simulink model "SimForces2022a"  (R2022a)
settings: Solver=daessc  StartTime=0.0  StopTime=10  FixedStep=0.001  RelTol=1e-4
values from neighbouring files (symbols this model uses):
  Bc1_V = [0;0;0;0;0;0]    [initializeSimulationGP.m]
  D22F = [0;0;0;0;0;0]    [initializeSimulationGP.m]
  filtDV = init2ndOrderLowPassFilter(35*2*pi,1,controller.dT)    [initializeLowPassFilters.m]
  filtEnc = init2ndOrderLowPassFilter(35*2*pi,1,controller.dT)    [initializeLowPassFilters.m]
undefined symbols (not defined in the file or in its folder): aux, B11_r_B11Tc1, B11_V, B11Ftot, B12_r_B12Tc2, B12_Rot_Tc2, B12_U_Tc2, B12_V, B12Ftot, B31_r_B31B41, B31_V, B31FTot, B32_r_B32B42, B32_Rot_B42, B32_U_B42, B32_V, B32FTot, B41_r_B41Tc1, B41_V, B41FTot, B42_r_B42Tc2, B42_Rot_Tc2, B42_U_Tc2, B42_V, B42FTot, B52_r_B52P32, B52_Rot_P32, B52_U_P32, B52_V, B52Ftot, Bc1_r_Bc1B11, Bc1_r_Bc1B31, Bc1FTot, Bc2_r_Bc2B12, Bc2_r_Bc2B32, Bc2_Rot_B12, Bc2_Rot_B32, Bc2_U_B12, Bc2_U_B32, Bc2_V, Bc2Tot, controller, cyl1, cyl2, D22_V, dq1, dq11, dq12, dq2, dq21, dq22, dx1, dx2, dxt2, fc1, fc1r, fc2, fc2r, fct2, fct2r ... (+61)
libraries: sm_lib x32, nesl_utility x20
(part 1 of 7)
settings Model: Creator=liikaneh  LastModifiedBy=casey
settings SolverCC: AlgebraicLoopSolver=TrustRegion
settings OptimizationCC: DefaultParameterBehavior=Inlined  GainParamInheritBuiltInType=on  UseFloatMulNetSlope=on  InlineInvariantSignals=on  EfficientFloat2IntCast=on
settings DebuggingCC: ReadBeforeWriteMsg=DisableAll  WriteAfterWriteMsg=DisableAll  WriteAfterReadMsg=DisableAll  MultiTaskDSMMsg=none  UnconnectedInputMsg=warning  UnconnectedOutputMsg=warning  UnconnectedLineMsg=warning  SFMachineParentedDataDiag=warning  ArithmeticOperatorsInVariantConditions=warning
settings ModelReferenceCC: UpdateModelReferenceTargets=IfOutOfDate
settings SFSimCC: SFSimEcho=off  SimUseLocalCustomCode=off  CustomCodeUndefinedFunction=UseInterfaceOnly
settings RTWCC: RTWUseLocalCustomCode=off  BuildConfiguration=Faster Runs  DLArmComputeVersion=19.05
settings GRTTargetCC: MatFileLogging=off  SupportNonFinite=off
settings DiagnosticsConfigSet: SimMechanicsRigidlyBoundBlock=none

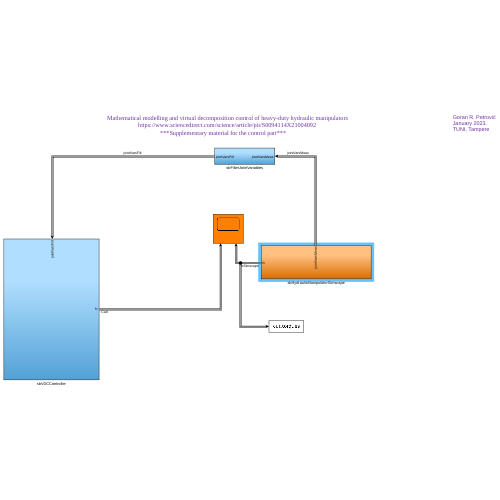
[thumbnail: Simulink's stored preview of the top-level diagram]
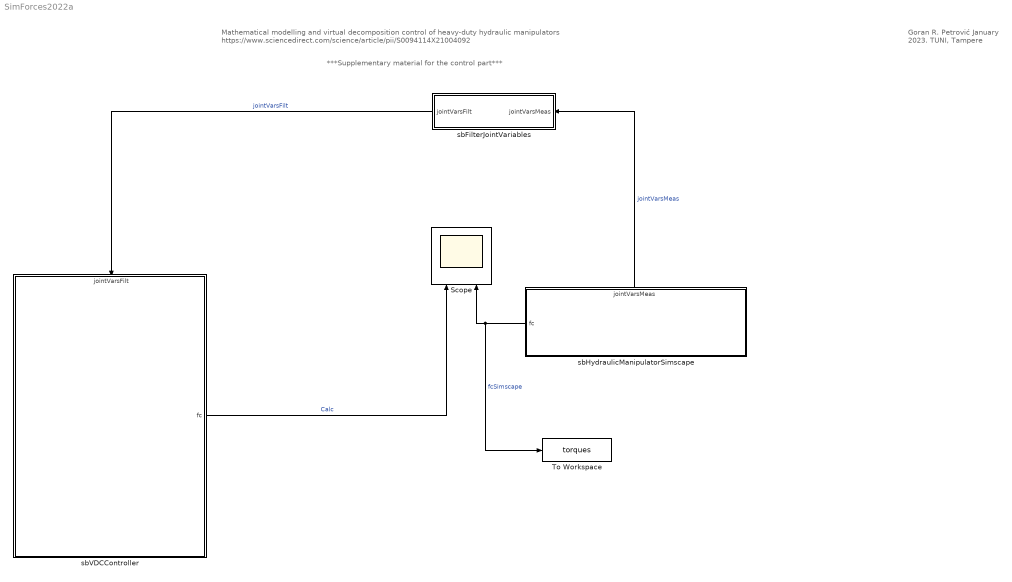
== system SimForces2022a ==
  note: ***Supplementary material for the control part***
  note: Mathematical modelling and virtual decomposition control of heavy-duty hydraulic manipulators
      | https://www.sciencedirect.com/science/article/pii/S0094114X21004092
  note: Goran R. Petrović
      | January 2023.
      | TUNI, Tampere
  Scope : Scope  NumInputPorts=2
  To Workspace : ToWorkspace  VariableName=torques  SaveFormat=Timeseries  SampleTime=-1
  sbFilterJointVariables : Subsystem
  sbHydraulicManipulatorSimscape : Subsystem
      settings: PortSchema="{\"entries\":[{\"content\":{\"sides\":[{\"content\":{\"connectorIds\":[\"Out2\"]},\"type\":\"ConnectorPlacement.EquallySpacedRectSide\",\"uuid\":\"f7b00952-2d51-484f-abea-a7edf7f1803a\"},{\"content\":{\"connectorIds\":[],\"side\":\"RIGHT\"},\"type\":\"ConnectorPlacement.EquallySpacedRectSide\",\"uuid\":\"cec57a8d-f407-43fc-b54f-695abbd67ebc\"},{\"content\":{\"connectorIds\":[\"Out1\"],\"side\":\"TOP\"},\"type\":\"ConnectorPlacement.EquallySpacedRectSide\",\"uuid\":\"36c8b0b2-f27a-4d8c-8e2c-18a80d711d3e\"}]},\"type\":\"ConnectorPlacement.EquallySpacedConnector\",\"uuid\":\"9ce8286e-5e91-4ec7-b364-968722180a48\"}],\"packageUris\":[\"http://schema.mathworks.com/mf0/Connector/R2020b\"],\"version\":\"1.0\"}"
  sbVDCController : Subsystem
      settings: PortSchema="{\"entries\":[{\"content\":{\"sides\":[{\"content\":{\"connectorIds\":[]},\"type\":\"ConnectorPlacement.EquallySpacedRectSide\",\"uuid\":\"7b05da7d-8e98-4260-b965-883aeff80f6d\"},{\"content\":{\"connectorIds\":[\"Out1\"],\"side\":\"RIGHT\"},\"type\":\"ConnectorPlacement.EquallySpacedRectSide\",\"uuid\":\"bab503f6-0cf2-4d25-8612-166524dadf44\"},{\"content\":{\"connectorIds\":[\"In1\"],\"side\":\"TOP\"},\"type\":\"ConnectorPlacement.EquallySpacedRectSide\",\"uuid\":\"dc9bf139-dfcc-4316-b9ab-c299ea19db13\"}]},\"type\":\"ConnectorPlacement.EquallySpacedConnector\",\"uuid\":\"a723f5e0-c36b-4f3a-b452-df4ada5825ab\"}],\"packageUris\":[\"http://schema.mathworks.com/mf0/Connector/R2020b\"],\"version\":\"1.0\"}"
  wires:
  sbHydraulicManipulatorSimscape/1(jointVarsMeas) -> sbFilterJointVariables/1(jointVarsMeas)  "jointVarsMeas"
  sbFilterJointVariables/1(jointVarsFilt) -> sbVDCController/1(jointVarsFilt)  "jointVarsFilt"
  sbVDCController/1(fc) -> Scope/1  "Calc"
  sbHydraulicManipulatorSimscape/2(fc) -> To Workspace/1, Scope/2  "fcSimscape"

== system SimForces2022a/sbFilterJointVariables ==
  jointVarsMeas : Inport  OutDataTypeStr=double  PortDimensions=3  SampleTime=controller.dT
  Bus Creator : BusCreator  Inputs=theta1Filt,theta2Filt,xt2Filt
  Bus Selector : BusSelector  OutputSignals=theta1Meas,theta2Meas,xt2Meas
  sbTheta1LowPassFilter : Subsystem
  sbTheta2LowPassFilter : Subsystem
  sbxt2LowPassFilter : Subsystem
  jointVarsFilt : Outport  OutDataTypeStr=double  PortDimensions=3  SampleTime=controller.dT
  wires:
  sbxt2LowPassFilter/1(xt2Filt) -> Bus Creator/3  "xt2Filt"
  sbTheta2LowPassFilter/1(theta2Filt) -> Bus Creator/2  "theta2Filt"
  sbTheta1LowPassFilter/1(theta1Filt) -> Bus Creator/1  "theta1Filt"
  Bus Selector/2 -> sbTheta2LowPassFilter/1(theta2Meas)  "<theta2Meas>"
  Bus Selector/1 -> sbTheta1LowPassFilter/1(theta1Meas)  "<theta1Meas>"
  Bus Selector/3 -> sbxt2LowPassFilter/1(xt2Meas)  "<xt2Meas>"
  jointVarsMeas/1 -> Bus Selector/1
  Bus Creator/1 -> jointVarsFilt/1

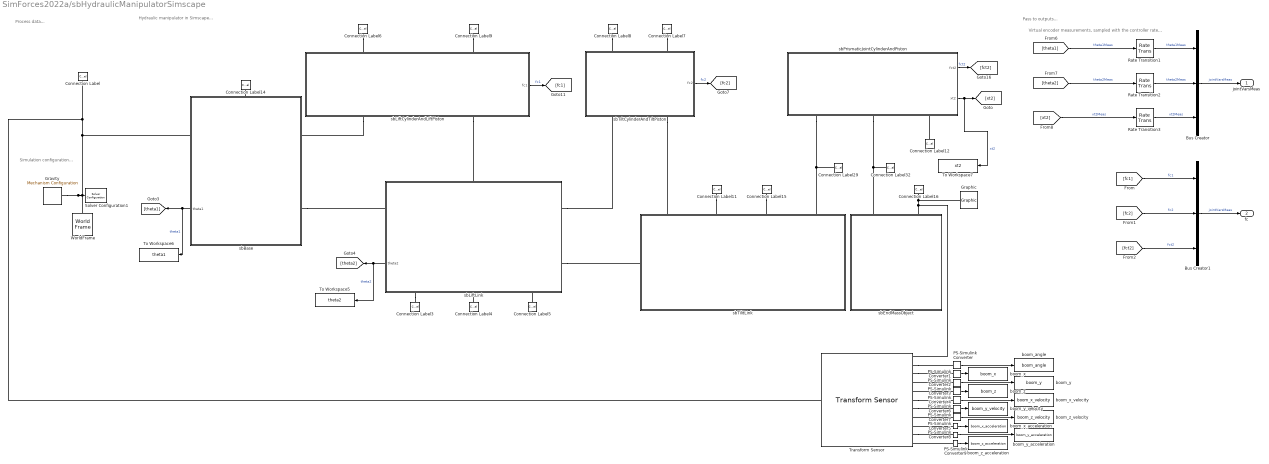
== system SimForces2022a/sbHydraulicManipulatorSimscape ==
  note: Process data...
  note: Hydraulic manipulator in Simscape...
  note: Simulation configuration...
  note: Pass to outputs...
  note: Virtual encoder measurements, sampled with the controller rate...
  Bus Creator : BusCreator  Inputs=theta1Meas,theta2Meas,xt2Meas
  Bus Creator1 : BusCreator  Inputs=fc1,fc2,fct2
  Connection Label : ConnectionLabel  Label=W
  Connection Label11 : ConnectionLabel  Label=B12
  Connection Label12 : ConnectionLabel  Label=B52
  Connection Label14 : ConnectionLabel  Label=Bc1
  Connection Label15 : ConnectionLabel  Label=Tc2
  Connection Label16 : ConnectionLabel  Label=D22
  Connection Label29 : ConnectionLabel  Label=P22
  Connection Label3 : ConnectionLabel  Label=Tc1
  Connection Label32 : ConnectionLabel  Label=P32
  Connection Label4 : ConnectionLabel  Label=B11
  Connection Label5 : ConnectionLabel  Label=Bc2
  Connection Label6 : ConnectionLabel  Label=B31
  Connection Label7 : ConnectionLabel  Label=B42
  Connection Label8 : ConnectionLabel  Label=B32
  Connection Label9 : ConnectionLabel  Label=B41
  Graphic : sm_lib/Body Elements/Graphic  GraphicType=Marker  MarkerShape=Frame  MarkerSize=50  GraphicVisPropType=SimpleVisualProperties  GraphicDiffuseColor=[0.9294 0.6941 0.1255]  GraphicSpecularColor=[0.5 0.5 0.5 1.0]  GraphicAmbientColor=[0.15 0.15 0.15 1.0]  GraphicEmissiveColor=[0.0 0.0 0.0 1.0]  GraphicShininess=75  GraphicOpacity=1.0
  Gravity : sm_lib/Utilities/Mechanism Configuration  UniformGravity=Constant  GravityVector=-gravity.Wg  GravityUnits=m/s^2  LinearizationDelta=0.001  JointModeTransitionNonlinearIterations=2
  PS-Simulink Converter{,1..9} (10 alike) : nesl_utility/PS-Simulink Converter  PhysicalDomain=network_engine_domain  SubClassName=ps_output  LeftPortType=input  RightPortType=output  PseudoPeriodic=off  Frequencies=[]  VectorFormat=inherit  Unit=inherit  AffineConversion=off
      settings: SourceProductBaseCode=SS,PW,VE
  Rate Transition1 : RateTransition  InitialCondition=initVals.theta10  OutPortSampleTime=controller.dT
  Rate Transition2 : RateTransition  InitialCondition=initVals.theta20  OutPortSampleTime=controller.dT
  Rate Transition3 : RateTransition  InitialCondition=initVals.xt20  OutPortSampleTime=controller.dT
  Solver Configuration1 : nesl_utility/Solver Configuration  PhysicalDomain=network_engine_domain  SubClassName=solver  LeftPortType=input  RightPortType=generic  Tones=[]  Harmonics=[]  SimulateNoise=off  Profile=off  UseLocalSampling=off  EnableSwitchedLinearOptims=on  FrequencyDomain=off  UseCCode=off  RelTol=0.001  AbsTol=1e-06  MinStep=1e-09  ToWorkspace=off  RevertToSquareIcSolve=off  NumHomotopyIterations=100  PhasorMode=off  PhasorModeNumHarmonics=1  IndexReductionMethod=DerivativeReplacement  DoDC=on  ResidualTolerance=1e-9  UseLocalSolver=off  LocalSolverChoice=NE_TRAPEZOIDAL_ADVANCER  LocalSolverSampleTime=0.002  DoFixedCost=off  MaxNonlinIter=3  MaxModeIter=2  ComputeImpulses=off  ImpulseIterations=2  LinearAlgebra=Sparse  LinearAlgebraNumThread=0  EquationFormulation=NE_TIME_EF  DelaysMemoryBudget=1024  AutomaticFiltering=on  FilteringTimeConstant=0.001  PartitionStorageMethod=AS_NEEDED  PartitionMemoryBudget=1024  PartitionMethod=FAST
      settings: SourceProductBaseCode=SS,PW,VE
  To Workspace5 : ToWorkspace  VariableName=theta2  SaveFormat=Timeseries  SampleTime=-1
  To Workspace6 : ToWorkspace  VariableName=theta1  SaveFormat=Timeseries  SampleTime=-1
  To Workspace7 : ToWorkspace  VariableName=xt2  SaveFormat=Timeseries  SampleTime=-1
  Transform Sensor : sm_lib/Frames and Transforms/Transform Sensor  MeasurementFrame=World  SenseAngle=on  SenseAxis=off  SenseAngle1=off  SenseAngle2=off  SenseAngle3=off  SenseQ=off  SenseR=off  SenseOmegaX=off  SenseOmegaY=off  SenseOmegaZ=off  SenseOmega1=off  SenseOmega2=off  SenseOmega3=off  SenseQDot=off  SenseRDot=off  SenseAlphaX=off  SenseAlphaY=off  SenseAlphaZ=off  SenseAlpha1=off  SenseAlpha2=off  SenseAlpha3=off  SenseQDDot=off  SenseRDDot=off  SenseX=on  SenseY=on  SenseZ=on  SenseRad=off  SenseAzim=off  SenseDist=off  SenseInc=off  SenseXDot=on  SenseYDot=on  SenseZDot=on  SenseRadDot=off  SenseAzimDot=off  SenseDistDot=off  SenseIncDot=off  SenseXDDot=on  SenseYDDot=on  SenseZDDot=on  SenseRadDDot=off  SenseAzimDDot=off  SenseDistDDot=off  SenseIncDDot=off
  WorldFrame : sm_lib/Frames and Transforms/World Frame
  boom_angle : ToWorkspace  VariableName=boom_angle  SaveFormat=Structure  SampleTime=-1
      settings: Save2DSignal=2-D array (concatenate along first dimension)
  boom_x : ToWorkspace  VariableName=boom_x  SaveFormat=Structure With Time  SampleTime=-1
  boom_x_acceleration : ToWorkspace  VariableName=boom_x_acceleration  SaveFormat=Structure  SampleTime=-1
      settings: Save2DSignal=2-D array (concatenate along first dimension)
  boom_x_velocity : ToWorkspace  VariableName=boom_x_velocity  SaveFormat=Structure  SampleTime=-1
      settings: Save2DSignal=2-D array (concatenate along first dimension)
  boom_y : ToWorkspace  VariableName=boom_y  SaveFormat=Structure  SampleTime=-1
      settings: Save2DSignal=2-D array (concatenate along first dimension)
  boom_y_acceleration : ToWorkspace  VariableName=boom_y_acceleration  SaveFormat=Structure  SampleTime=-1
      settings: Save2DSignal=2-D array (concatenate along first dimension)
  boom_y_velocity : ToWorkspace  VariableName=boom_y_velocity  SaveFormat=Structure  SampleTime=-1
      settings: Save2DSignal=2-D array (concatenate along first dimension)
  boom_z : ToWorkspace  VariableName=boom_z  SaveFormat=Structure  SampleTime=-1
      settings: Save2DSignal=2-D array (concatenate along first dimension)
  boom_z_acceleration : ToWorkspace  VariableName=boom_z_acceleration  SaveFormat=Structure  SampleTime=-1
      settings: Save2DSignal=2-D array (concatenate along first dimension)
  boom_z_velocity : ToWorkspace  VariableName=boom_z_velocity  SaveFormat=Structure  SampleTime=-1
      settings: Save2DSignal=2-D array (concatenate along first dimension)
  sbBase : Subsystem
      settings: PortSchema="{\"entries\":[{\"content\":{\"sides\":[{\"content\":{\"connectorIds\":[\"LConn1\",\"Out1\"]},\"type\":\"ConnectorPlacement.EquallySpacedRectSide\",\"uuid\":\"74e7f3c6-cbce-4102-a556-47a2132f5eea\"},{\"content\":{\"connectorIds\":[\"RConn1\",\"RConn2\"],\"side\":\"RIGHT\"},\"type\":\"ConnectorPlacement.EquallySpacedRectSide\",\"uuid\":\"9dc74751-c8ff-4cb6-874a-dcd58e00de96\"},{\"content\":{\"connectorIds\":[\"LConn2\"],\"side\":\"TOP\"},\"type\":\"ConnectorPlacement.EquallySpacedRectSide\",\"uuid\":\"06e145de-a8a9-4531-940d-434d89c78f5b\"}]},\"type\":\"ConnectorPlacement.EquallySpacedConnector\",\"uuid\":\"f796a1f4-9531-411f-8f55-fdef488b8a52\"}],\"packageUris\":[\"http://schema.mathworks.com/mf0/Connector/R2020b\"],\"version\":\"1.0\"}"
  sbEndMassObject : Subsystem
      settings: PortSchema="{\"entries\":[{\"content\":{\"sides\":[{\"content\":{\"connectorIds\":[]},\"type\":\"ConnectorPlacement.EquallySpacedRectSide\",\"uuid\":\"c1652833-a888-40a4-a60e-17be9708feae\"},{\"content\":{\"connectorIds\":[],\"side\":\"RIGHT\"},\"type\":\"ConnectorPlacement.EquallySpacedRectSide\",\"uuid\":\"55671429-adc4-418e-b6f5-c624f049c776\"},{\"content\":{\"connectorIds\":[\"LConn1\",\"LConn2\"],\"side\":\"TOP\"},\"type\":\"ConnectorPlacement.EquallySpacedRectSide\",\"uuid\":\"549e793d-1b28-4f93-9706-f4524b8bc4e2\"}]},\"type\":\"ConnectorPlacement.EquallySpacedConnector\",\"uuid\":\"9a6e434f-5824-411f-a3a4-9b8ec603a501\"}],\"packageUris\":[\"http://schema.mathworks.com/mf0/Connector/19700101\"],\"version\":\"1.0\"}"
  sbLiftCylinderAndLiftPiston : Subsystem
      settings: PortSchema="{\"entries\":[{\"content\":{\"sides\":[{\"content\":{\"connectorIds\":[]},\"type\":\"ConnectorPlacement.EquallySpacedRectSide\",\"uuid\":\"a609877c-275e-4024-96c6-67831631fbf9\"},{\"content\":{\"connectorIds\":[\"Out1\"],\"side\":\"RIGHT\"},\"type\":\"ConnectorPlacement.EquallySpacedRectSide\",\"uuid\":\"b747ace3-04d7-42f4-87a7-c62fd6093e0d\"},{\"content\":{\"connectorIds\":[\"LConn1\",\"LConn2\"],\"side\":\"TOP\"},\"type\":\"ConnectorPlacement.EquallySpacedRectSide\",\"uuid\":\"5f9db8d6-814e-4333-b197-0e9dcf847d3e\"},{\"content\":{\"connectorIds\":[\"RConn1\",\"RConn2\"],\"side\":\"BOTTOM\"},\"type\":\"ConnectorPlacement.EquallySpacedRectSide\",\"uuid\":\"d1d564c3-4146-4330-9936-8dd25e0cb4bf\"}]},\"type\":\"ConnectorPlacement.EquallySpacedConnector\",\"uuid\":\"d00f43c3-717c-4aa5-b919-dd57ad6708f7\"}],\"packageUris\":[\"http://schema.mathworks.com/mf0/Connector/R2020b\"],\"version\":\"1.0\"}"
  sbLiftLink : Subsystem
      settings: PortSchema="{\"entries\":[{\"content\":{\"sides\":[{\"content\":{\"connectorIds\":[\"LConn1\",\"LConn2\"]},\"type\":\"ConnectorPlacement.EquallySpacedRectSide\",\"uuid\":\"50668ed3-3246-41c6-a320-c5b34ebd86b6\"},{\"content\":{\"connectorIds\":[\"RConn1\",\"Out1\"],\"side\":\"RIGHT\"},\"type\":\"ConnectorPlacement.EquallySpacedRectSide\",\"uuid\":\"d76ddc23-e4dc-4bdf-9e15-3eadac6cf1e2\"},{\"content\":{\"connectorIds\":[\"LConn3\"],\"side\":\"TOP\"},\"type\":\"ConnectorPlacement.EquallySpacedRectSide\",\"uuid\":\"5458eee7-805c-4d74-888c-3f811d80880c\"},{\"content\":{\"connectorIds\":[\"RConn2\",\"RConn3\",\"RConn4\"],\"side\":\"BOTTOM\"},\"type\":\"ConnectorPlacement.EquallySpacedRectSide\",\"uuid\":\"6f630415-b321-44c9-a6f9-9daa6b5086dd\"}]},\"type\":\"ConnectorPlacement.EquallySpacedConnector\",\"uuid\":\"adbb0eba-5908-47e0-8cde-3ca3a2901b66\"}],\"packageUris\":[\"http://schema.mathworks.com/mf0/Connector/R2020b\"],\"version\":\"1.0\"}"
  sbPrismaticJointCylinderAndPiston : Subsystem
      settings: PortSchema="{\"entries\":[{\"content\":{\"sides\":[{\"content\":{\"connectorIds\":[]},\"type\":\"ConnectorPlacement.EquallySpacedRectSide\",\"uuid\":\"002196eb-b81c-4ad4-9df1-33c4ef5d5c77\"},{\"content\":{\"connectorIds\":[\"Out1\",\"Out2\"],\"side\":\"RIGHT\"},\"type\":\"ConnectorPlacement.EquallySpacedRectSide\",\"uuid\":\"e0d61efe-ea5d-4756-bea5-1d107b09975a\"},{\"content\":{\"connectorIds\":[],\"side\":\"TOP\"},\"type\":\"ConnectorPlacement.EquallySpacedRectSide\",\"uuid\":\"1a952641-c922-4f91-9854-1cf1d6e715db\"},{\"content\":{\"connectorIds\":[\"RConn1\",\"RConn2\",\"RConn3\"],\"side\":\"BOTTOM\"},\"type\":\"ConnectorPlacement.EquallySpacedRectSide\",\"uuid\":\"13c3128f-85d9-4df5-9ae2-f45a9cb5a20e\"}]},\"type\":\"ConnectorPlacement.EquallySpacedConnector\",\"uuid\":\"7bd12321-8448-494e-b8ce-fe2f63fec7f7\"}],\"packageUris\":[\"http://schema.mathworks.com/mf0/Connector/R2020b\"],\"version\":\"1.0\"}"
  sbTilitLink : Subsystem
      settings: PortSchema="{\"entries\":[{\"content\":{\"sides\":[{\"content\":{\"connectorIds\":[]},\"type\":\"ConnectorPlacement.EquallySpacedRectSide\",\"uuid\":\"3124f0ed-3daa-4e61-aa81-877c0a0fd3a0\"},{\"content\":{\"connectorIds\":[\"RConn1\"],\"side\":\"RIGHT\"},\"type\":\"ConnectorPlacement.EquallySpacedRectSide\",\"uuid\":\"bc27bd78-7de5-476c-8b4b-17e2ed4c2476\"},{\"content\":{\"connectorIds\":[\"LConn1\",\"LConn2\",\"LConn3\",\"LConn4\"],\"side\":\"TOP\"},\"type\":\"ConnectorPlacement.EquallySpacedRectSide\",\"uuid\":\"46b542cf-bb62-4410-9418-b726c84ee3f9\"}]},\"type\":\"ConnectorPlacement.EquallySpacedConnector\",\"uuid\":\"3938a7f2-fa69-42c9-abcf-1c8c25e9b66f\"}],\"packageUris\":[\"http://schema.mathworks.com/mf0/Connector/19700101\"],\"version\":\"1.0\"}"
  sbTiltCylinderAndTiltPiston : Subsystem
      settings: PortSchema="{\"entries\":[{\"content\":{\"sides\":[{\"content\":{\"connectorIds\":[]},\"type\":\"ConnectorPlacement.EquallySpacedRectSide\",\"uuid\":\"a609877c-275e-4024-96c6-67831631fbf9\"},{\"content\":{\"connectorIds\":[\"Out1\"],\"side\":\"RIGHT\"},\"type\":\"ConnectorPlacement.EquallySpacedRectSide\",\"uuid\":\"b747ace3-04d7-42f4-87a7-c62fd6093e0d\"},{\"content\":{\"connectorIds\":[\"LConn1\",\"LConn2\"],\"side\":\"TOP\"},\"type\":\"ConnectorPlacement.EquallySpacedRectSide\",\"uuid\":\"5f9db8d6-814e-4333-b197-0e9dcf847d3e\"},{\"content\":{\"connectorIds\":[\"RConn1\",\"RConn2\"],\"side\":\"BOTTOM\"},\"type\":\"ConnectorPlacement.EquallySpacedRectSide\",\"uuid\":\"d1d564c3-4146-4330-9936-8dd25e0cb4bf\"}]},\"type\":\"ConnectorPlacement.EquallySpacedConnector\",\"uuid\":\"d00f43c3-717c-4aa5-b919-dd57ad6708f7\"}],\"packageUris\":[\"http://schema.mathworks.com/mf0/Connector/R2020b\"],\"version\":\"1.0\"}"
  jointVarsMeas : Outport
  fc : Outport  Port=2
  wires:
  sbLiftCylinderAndLiftPiston/1(fc1) -> [fc1]  "fc1"
  sbTiltCylinderAndTiltPiston/1(fc2) -> [fc2]  "fc2"
  sbPrismaticJointCylinderAndPiston/1(fct2) -> [fct2]  "fct2"
  sbLiftLink/1(theta2) -> [theta2], To Workspace5/1  "theta2"
  sbBase/1(theta1) -> To Workspace6/1, [theta1]  "theta1"
  Bus Creator/1 -> jointVarsMeas/1  "jointVarsMeas"
  [theta2] -> Rate Transition2/1  "theta2Meas"
  Rate Transition1/1 -> Bus Creator/1  "theta1Meas"
  Rate Transition2/1 -> Bus Creator/2  "theta2Meas"
  Rate Transition3/1 -> Bus Creator/3  "xt2Meas"
  [theta1] -> Rate Transition1/1  "theta1Meas"
  [xt2] -> Rate Transition3/1  "xt2Meas"
  [fc1] -> Bus Creator1/1  "fc1"
  [fc2] -> Bus Creator1/2  "fc2"
  [fct2] -> Bus Creator1/3  "fct2"
  Bus Creator1/1 -> fc/1  "jointVarsMeas"
  sbPrismaticJointCylinderAndPiston/2(xt2) -> To Workspace7/1, [xt2]  "xt2"
  PS-Simulink Converter4/1 -> boom_x_velocity/1
  PS-Simulink Converter3/1 -> boom_z/1
  PS-Simulink Converter/1 -> boom_angle/1
  PS-Simulink Converter1/1 -> boom_x/1
  PS-Simulink Converter2/1 -> boom_y/1
  PS-Simulink Converter6/1 -> boom_y_velocity/1
  PS-Simulink Converter5/1 -> boom_x_acceleration/1
  PS-Simulink Converter7/1 -> boom_z_velocity/1
  PS-Simulink Converter8/1 -> boom_y_acceleration/1
  PS-Simulink Converter9/1 -> boom_z_acceleration/1
  connections:
  Gravity/RConn1 -- sbBase/LConn1 -- Connection Label/LConn1 -- Transform Sensor/LConn1 -- WorldFrame/RConn1 -- Solver Configuration1/RConn1
  sbLiftLink/LConn1 -- sbTiltCylinderAndTiltPiston/RConn1
  sbLiftLink/LConn2 -- sbTilitLink/RConn1
  sbTiltCylinderAndTiltPiston/RConn2 -- sbTilitLink/LConn4
  sbLiftCylinderAndLiftPiston/RConn2 -- sbLiftLink/LConn3
  sbBase/RConn2 -- sbLiftLink/RConn1
  sbLiftCylinderAndLiftPiston/RConn1 -- sbBase/RConn1
  sbLiftLink/RConn4 -- Connection Label3/LConn1
  Connection Label4/LConn1 -- sbLiftLink/RConn3
  Connection Label5/LConn1 -- sbLiftLink/RConn2
  Connection Label6/LConn1 -- sbLiftCylinderAndLiftPiston/LConn1
  Connection Label9/LConn1 -- sbLiftCylinderAndLiftPiston/LConn2
  Connection Label7/LConn1 -- sbTiltCylinderAndTiltPiston/LConn2
  Connection Label8/LConn1 -- sbTiltCylinderAndTiltPiston/LConn1
  Connection Label11/LConn1 -- sbTilitLink/LConn3
  Connection Label15/LConn1 -- sbTilitLink/LConn2
  Connection Label16/LConn1 -- Graphic/RConn1 -- sbEndMassObject/LConn2 -- Transform Sensor/RConn1
  Connection Label14/LConn1 -- sbBase/LConn2
  Connection Label12/LConn1 -- sbPrismaticJointCylinderAndPiston/RConn3
  sbPrismaticJointCylinderAndPiston/RConn1 -- Connection Label29/LConn1 -- sbTilitLink/LConn1
  sbPrismaticJointCylinderAndPiston/RConn2 -- sbEndMassObject/LConn1 -- Connection Label32/LConn1
  Transform Sensor/RConn2 -- PS-Simulink Converter/LConn1
  Transform Sensor/RConn3 -- PS-Simulink Converter1/LConn1
  PS-Simulink Converter2/LConn1 -- Transform Sensor/RConn4
  Transform Sensor/RConn6 -- PS-Simulink Converter4/LConn1
  PS-Simulink Converter3/LConn1 -- Transform Sensor/RConn5
  PS-Simulink Converter5/LConn1 -- Transform Sensor/RConn9
  Transform Sensor/RConn7 -- PS-Simulink Converter6/LConn1
  PS-Simulink Converter7/LConn1 -- Transform Sensor/RConn8
  Transform Sensor/RConn10 -- PS-Simulink Converter8/LConn1
  PS-Simulink Converter9/LConn1 -- Transform Sensor/RConn11

== system SimForces2022a/sbVDCController ==
  note: Extract actuator forces per (73) and (76).
  note: Forming total forces.
  note: Geometric relations (18) - (23), velocities (24) - (34), along with all the necessary rotation matrices and force/velocity
      | transformation matrices (5) are formed here.
  note: Calculate qj angles as they are starting point for kinematic relations (18) - (23).
  note: Required piston forces for comparison puroposes...
  note: Select from existing buses...
  note: No required force imposing on the surroundings...
  note: Zero-vector for a fixed base....
  note: Filtered values of joint variables...
  note: Process data...
  note: Get inputs...
  note: Pass to outputs...
  jointVarsFilt : Inport
  Bus Selector : BusSelector  OutputSignals=theta1Filt,theta2Filt,xt2Filt
  Constant1 : Constant  Value=Bc1_V
  D22F : Constant  Value=D22F
  Rate Transition : RateTransition  OutPortSampleTime=controller.dT
  sbAuxiliaryJointAngles : Subsystem
  sbCalculateRequiredActuatorForces : Subsystem
  sbFormAnalyticQuantities : Subsystem
  sbFormTotalRequiredForces : Subsystem
  fc : Outport
  wires:
  Bus Selector/3 -> [xt2Filt]  "<xt2Filt>"
  Bus Selector/2 -> [theta2Filt]  "<theta2Filt>"
  [Bc1V] -> sbFormAnalyticQuantities/4(Bc1V)  "Bc1V"
  [D22F] -> sbCalculateRequiredActuatorForces/4(D22F)  "D22F"
  sbAuxiliaryJointAngles/1(q1) -> [q1]  "q1"
  [xt2Filt] -> sbFormAnalyticQuantities/3(xt2Filt)  "xt2Filt"
  [jointVarsFilt] -> Bus Selector/1  "jointVarsFilt"
  [WRotX] -> sbFormTotalRequiredForces/2(WRotX)  "WRotX"
  sbFormTotalRequiredForces/1(FTotX) -> [FTotX]  "FTotX"
  [velsX] -> sbFormTotalRequiredForces/1(velsX)  "velsX"
  [FTotX] -> sbCalculateRequiredActuatorForces/1(FTotX)  "FTotX"
  [geomPropX] -> sbCalculateRequiredActuatorForces/3(geomPropX)  "geomPropX"
  Constant1/1 -> [Bc1V]  "Bc1_V"
  sbFormAnalyticQuantities/3(UMatsX) -> [UMatsX]  "UMatsX"
  sbFormAnalyticQuantities/1(geomPropX) -> [geomPropX]  "geomPropX"
  [theta2Filt] -> sbAuxiliaryJointAngles/2(theta2Filt)  "theta2Filt"
  [theta1Filt] -> sbAuxiliaryJointAngles/1(theta1Filt)  "theta1Filt"
  sbFormAnalyticQuantities/2(WRotX) -> [WRotX]  "WRotX"
  D22F/1 -> [D22F]  "D22F"
  [UMatsX] -> sbCalculateRequiredActuatorForces/2(UMatsX)  "UMatsX"
  [q2] -> sbFormAnalyticQuantities/2(q2)  "q2"
  [q1] -> sbFormAnalyticQuantities/1(q1)  "q1"
  sbAuxiliaryJointAngles/2(q2) -> [q2]  "q2"
  sbFormAnalyticQuantities/4(velsX) -> [velsX]  "velsX"
  Bus Selector/1 -> [theta1Filt]  "<theta1Filt>"
  jointVarsFilt/1 -> [jointVarsFilt]  "jointVarsFilt"
  sbCalculateRequiredActuatorForces/1(fcr) -> [fc]  "fc"
  [fc] -> Rate Transition/1  "fc"
  Rate Transition/1 -> fc/1  "fc"

== system SimForces2022a/sbFilterJointVariables/sbTheta1LowPassFilter ==
  theta1Meas : Inport
  Delay : Delay  InitialConditionSource=Input port  SampleTime=filtEnc.dT
      settings: InputPortMap=u0,p4
  Delay1 : Delay  DelayLength=1  InitialConditionSource=Input port  SampleTime=filtEnc.dT
      settings: InputPortMap=u0,p4
  Delay2 : Delay  DelayLength=0  InitialConditionSource=Input port  SampleTime=filtEnc.dT
      settings: InputPortMap=u0,p4
  Delay3 : Delay  InitialConditionSource=Input port  SampleTime=filtEnc.dT
      settings: InputPortMap=u0,p4
  Delay4 : Delay  DelayLength=1  InitialConditionSource=Input port  SampleTime=filtEnc.dT
      settings: InputPortMap=u0,p4
  Gain : Gain  Gain=filtEnc.a0
  Gain1 : Gain  Gain=filtEnc.b1
  Gain2 : Gain  Gain=filtEnc.b2
  Gain3 : Gain  Gain=filtEnc.b0
  Gain4 : Gain  Gain=filtEnc.a1
  Sum : Sum  Inputs=|--+++
  theta1Filt : Outport
  wires:
  Gain3/1 -> Sum/5
  Sum/1 -> theta1Filt/1, Delay4/1, Delay/1  "theta1Filt"
  Delay2/1 -> Gain2/1
  Delay/1 -> Gain/1
  Delay1/1 -> Gain1/1
  Gain4/1 -> Sum/1
  Delay4/1 -> Gain4/1
  Gain2/1 -> Sum/3
  theta1Meas/1 -> Delay4/2, Delay/2, Delay2/1, Delay2/2, Delay1/1, Delay3/2, Delay3/1, Delay1/2  "theta1Meas"
  Delay3/1 -> Gain3/1
  Gain/1 -> Sum/2
  Gain1/1 -> Sum/4

== system SimForces2022a/sbFilterJointVariables/sbTheta2LowPassFilter ==
  theta2Meas : Inport
  Delay : Delay  InitialConditionSource=Input port  SampleTime=filtEnc.dT
      settings: InputPortMap=u0,p4
  Delay1 : Delay  DelayLength=1  InitialConditionSource=Input port  SampleTime=filtEnc.dT
      settings: InputPortMap=u0,p4
  Delay2 : Delay  DelayLength=0  InitialConditionSource=Input port  SampleTime=filtEnc.dT
      settings: InputPortMap=u0,p4
  Delay3 : Delay  InitialConditionSource=Input port  SampleTime=filtEnc.dT
      settings: InputPortMap=u0,p4
  Delay4 : Delay  DelayLength=1  InitialConditionSource=Input port  SampleTime=filtEnc.dT
      settings: InputPortMap=u0,p4
  Gain : Gain  Gain=filtEnc.a0
  Gain1 : Gain  Gain=filtEnc.b1
  Gain2 : Gain  Gain=filtEnc.b2
  Gain3 : Gain  Gain=filtEnc.b0
  Gain4 : Gain  Gain=filtEnc.a1
  Sum : Sum  Inputs=|--+++
  theta2Filt : Outport
  wires:
  Gain3/1 -> Sum/5
  Gain2/1 -> Sum/3
  Delay4/1 -> Gain4/1
  Delay/1 -> Gain/1
  Delay1/1 -> Gain1/1
  Delay2/1 -> Gain2/1
  Gain4/1 -> Sum/1
  Sum/1 -> theta2Filt/1, Delay4/1, Delay/1  "theta2Filt"
  Gain1/1 -> Sum/4
  Gain/1 -> Sum/2
  Delay3/1 -> Gain3/1
  theta2Meas/1 -> Delay4/2, Delay/2, Delay2/1, Delay2/2, Delay1/1, Delay3/2, Delay3/1, Delay1/2  "theta2Meas"

== system SimForces2022a/sbFilterJointVariables/sbxt2LowPassFilter ==
  xt2Meas : Inport
  Delay : Delay  InitialConditionSource=Input port  SampleTime=filtEnc.dT
      settings: InputPortMap=u0,p4
  Delay1 : Delay  DelayLength=1  InitialConditionSource=Input port  SampleTime=filtEnc.dT
      settings: InputPortMap=u0,p4
  Delay2 : Delay  DelayLength=0  InitialConditionSource=Input port  SampleTime=filtEnc.dT
      settings: InputPortMap=u0,p4
  Delay3 : Delay  InitialConditionSource=Input port  SampleTime=filtEnc.dT
      settings: InputPortMap=u0,p4
  Delay4 : Delay  DelayLength=1  InitialConditionSource=Input port  SampleTime=filtEnc.dT
      settings: InputPortMap=u0,p4
  Gain : Gain  Gain=filtEnc.a0
  Gain1 : Gain  Gain=filtEnc.b1
  Gain2 : Gain  Gain=filtEnc.b2
  Gain3 : Gain  Gain=filtEnc.b0
  Gain4 : Gain  Gain=filtEnc.a1
  Sum : Sum  Inputs=|--+++
  xt2Filt : Outport
  wires:
  Gain/1 -> Sum/2
  xt2Meas/1 -> Delay2/1, Delay2/2, Delay1/1, Delay3/2, Delay3/1, Delay1/2, Delay4/2, Delay/2  "xt2Meas"
  Delay2/1 -> Gain2/1
  Sum/1 -> xt2Filt/1, Delay4/1, Delay/1  "xt2Filt"
  Gain4/1 -> Sum/1
  Gain2/1 -> Sum/3
  Gain3/1 -> Sum/5
  Delay1/1 -> Gain1/1
  Delay3/1 -> Gain3/1
  Delay/1 -> Gain/1
  Delay4/1 -> Gain4/1
  Gain1/1 -> Sum/4

== system SimForces2022a/sbHydraulicManipulatorSimscape/sbBase ==
  note: Defines world (W) frame.
  note: Resembles an ideal encoder.
  BaseR_To_W : sm_lib/Frames and Transforms/Rigid Transform  TranslationMethod=None  TranslationStandardOffset=0  TranslationLengthUnit=m  TranslationStandardAxis=+Z  TranslationCartesianOffset=[0 0 0]  TranslationROffset=0  TranslationROffsetUnits=m  TranslationZOffset=0  TranslationZOffsetUnits=m  TranslationThetaOffset=0  TranslationThetaOffsetUnits=deg  RotationMethod=StandardAxis  RotationAngleUnits=deg  RotationStandardAxis=+Y  RotationAngle=90  RotationArbitraryAxis=[0 0 1]  FollAlignAxisA=+X  BaseAlignAxisA=+Y  FollAlignAxisB=+Y  BaseAlignAxisB=+Z  RotationSequenceAxes=FollowerAxes  RotationSequence=XYX  RotationSequenceAngles=[0 0 0]  RotationSequenceAnglesUnits=deg  RotationMatrix=[1 0 0; 0 1 0; 0 0 1]
  BaseSolid : sm_lib/Body Elements/File Solid  ExtGeomFileName=01_BaseGP.STEP  UnitType=FromFile  ExtGeomFileUnits=m  StepReaderType=OCC  ExportConvexHullGeometry=off  InertiaType=Custom  Mass=307.29601379  MassUnits=kg  CenterOfMass=[0 -0.01488967 0.02139206]  CenterOfMassUnits=m  MomentsOfInertia=[29.78955950 5.25917100 29.30269608]  MomentsOfInertiaUnits=kg*m^2  ProductsOfInertia=[-3.89461427 -0.00003008 -0.00000910]  ProductsOfInertiaUnits=kg*m^2  BasedOnType=Density  Density=7300  DensityUnits=kg/m^3  DoExposeReferenceFrame=on  SerializedFrames=<Frames><Frame><Id>Frame1</Id><Value><Name>F2</Name><Origin><Source>GeometricFeature</Source><FeatureName>cylindrical surface 2</FeatureName></Origin><PrimaryAxis><DefinedDirection>+X</DefinedDirection><Source>ReferenceFrame</Source><SourceDirection>-Z</SourceDirection><FeatureName></FeatureName></PrimaryAxis><SecondaryAxis><DefinedDirection>+Y</DefinedDirection><Source>ReferenceFrame</Source><SourceDirection>+Y</SourceDirection><FeatureName></FeatureName></SecondaryAxis></Value></Frame><Frame><Id>Frame2</Id><Value><Name>F1</Name><Origin><Source>GeometricFeature</Source><FeatureName>cylindrical surface 1</FeatureName></Origin><PrimaryAxis><DefinedDirection>-X</DefinedDirection><Source>ReferenceFrame</Source><SourceDirection>+Z</SourceDirection><FeatureName></FeatureName></PrimaryAxis><SecondaryAxis><DefinedDirection>+Y</DefinedDirection><Source>ReferenceFrame</Source><SourceDirection>+Y</SourceDirection><FeatureName></FeatureName></SecondaryAxis></Value></Frame><Frame><Id>Frame3</Id><Value><Name>Bc1</Name><Origin><Source>GeometricFeature</Source><FeatureName>cylindrical surface 1</FeatureName></Origin><PrimaryAxis><DefinedDirection>+X</DefinedDirection><Source>GeometricFeature</Source><SourceDirection>+Z</SourceDirection><FeatureName>segment 135</FeatureName></PrimaryAxis><SecondaryAxis><DefinedDirection>+Y</DefinedDirection><Source>ReferenceFrame</Source><SourceDirection>+Z</SourceDirection><FeatureName></FeatureName></SecondaryAxis></Value></Frame></Frames>  GraphicType=FromGeometry  MarkerShape=Sphere  MarkerSize=10  GraphicVisPropType=SimpleVisualProperties  GraphicDiffuseColor=[134 134 71]/255  GraphicSpecularColor=[0.5 0.5 0.5 1.0]  GraphicAmbientColor=[0.15 0.15 0.15 1.0]  GraphicEmissiveColor=[0.0 0.0 0.0 1.0]  GraphicShininess=75  GraphicOpacity=1.0
  PS-Simulink Converter : nesl_utility/PS-Simulink Converter  PhysicalDomain=network_engine_domain  SubClassName=ps_output  LeftPortType=input  RightPortType=output  PseudoPeriodic=off  Frequencies=[]  VectorFormat=inherit  Unit=inherit  AffineConversion=off
      settings: SourceProductBaseCode=SS,PW,VE
  Simulink-PS Converter : nesl_utility/Simulink-PS Converter  PhysicalDomain=network_engine_domain  SubClassName=ps_input  LeftPortType=input  RightPortType=output  PseudoPeriodic=off  Frequencies=[]  NoiseDistribution=none  NoiseParameters=[]  Unit=1  AffineConversion=off  FilteringAndDerivatives=filter  SimscapeFilterOrder=2  InputFilterTimeConstant=0.01  UdotUserProvided=0
      settings: SourceProductBaseCode=SS,PW,VE
  Sine Wave : Sin  Amplitude=-0.47044  Frequency=0.31807  Phase=-2.3925  SampleTime=0
  theta1Rotation : sm_lib/Joints/Revolute Joint  JointMode=Normal  SenseConstraintForce=off  SenseConstraintForceX=off  SenseConstraintForceY=off  SenseConstraintForceZ=off  SenseConstraintTorque=off  SenseConstraintTorqueX=off  SenseConstraintTorqueY=off  SenseConstraintTorqueZ=off  SenseTotalForce=off  SenseTotalForceX=off  SenseTotalForceY=off  SenseTotalForceZ=off  SenseTotalTorque=off  SenseTotalTorqueX=off  SenseTotalTorqueY=off  SenseTotalTorqueZ=off  CompositeWrenchDir=FollowerOnBase  CompositeWrenchFrame=BaseFrame  EquilibriumPosition=0  EquilibriumPositionUnits=rad  SpringStiffness=0  SpringStiffnessUnits=N*m/rad  DampingCoefficient=0  DampingCoefficientUnits=N*m/(rad/s)  TorqueActuationMode=NoTorque  MotionActuationMode=InputMotion  SensePosition=on  SenseVelocity=off  SenseAcceleration=off  SenseTorqueForce=off  SenseLowerLimitTorqueForce=off  SenseUpperLimitTorqueForce=off  LowerLimitSpecify=off  LowerLimitBound=-90  LowerLimitBoundUnits=deg  LowerLimitStiffness=1e4  LowerLimitStiffnessUnits=N*m/deg  LowerLimitDamping=10  LowerLimitDampingUnits=N*m/(deg/s)  LowerLimitTransitionRegionWidth=0.1  LowerLimitTransitionRegionWidthUnits=deg  UpperLimitSpecify=off  UpperLimitBound=90  UpperLimitBoundUnits=deg  UpperLimitStiffness=1e4  UpperLimitStiffnessUnits=N*m/deg  UpperLimitDamping=10  UpperLimitDampingUnits=N*m/(deg/s)  UpperLimitTransitionRegionWidth=0.1  UpperLimitTransitionRegionWidthUnits=deg  PositionTargetSpecify=on  PositionTargetPriority=High  PositionTargetValue=initVals.theta10  PositionTargetValueUnits=rad  VelocityTargetSpecify=on  VelocityTargetPriority=High  VelocityTargetValue=0  VelocityTargetValueUnits=rad/s
  W : PMIOPort  Side=Left
  Bc1 : PMIOPort  Port=2  Side=Left
  F1 : PMIOPort  Port=3  Side=Right
  F2_rot : PMIOPort  Port=4  Side=Right
  theta1 : Outport
  wires:
  PS-Simulink Converter/1 -> theta1/1
  Sine Wave/1 -> Simulink-PS Converter/1
  connections:
  BaseR_To_W/LConn1 -- BaseSolid/RConn1
  W/RConn1 -- BaseR_To_W/RConn1
  theta1Rotation/LConn1 -- BaseSolid/LConn1
  F2_rot/RConn1 -- theta1Rotation/RConn1
  F1/RConn1 -- BaseSolid/LConn2
  Bc1/RConn1 -- BaseSolid/RConn2
  PS-Simulink Converter/LConn1 -- theta1Rotation/RConn2
  Simulink-PS Converter/RConn1 -- theta1Rotation/LConn2

== system SimForces2022a/sbHydraulicManipulatorSimscape/sbEndMassObject ==
  EndObjectMass : sm_lib/Body Elements/File Solid  ExtGeomFileName=10_ObjectGP.STEP  UnitType=FromFile  ExtGeomFileUnits=m  StepReaderType=OCC  ExportConvexHullGeometry=off  InertiaType=Custom  Mass=570.18877059  MassUnits=kg  CenterOfMass=[2.16142487 0.01347152 0.06601658]  CenterOfMassUnits=m  MomentsOfInertia=[46.81220713 72.19317437 67.11012925]  MomentsOfInertiaUnits=kg*m^2  ProductsOfInertia=[0.04641137 0.08825278 0.37588204]  ProductsOfInertiaUnits=kg*m^2  BasedOnType=Density  Density=7850  DensityUnits=kg/m^3  DoExposeReferenceFrame=off  SerializedFrames=<Frames><Frame><Id>Frame1</Id><Value><Name>P32p</Name><Origin><Source>GeometricFeature</Source><FeatureName>circular curve 7</FeatureName></Origin><PrimaryAxis><DefinedDirection>+Y</DefinedDirection><Source>GeometricFeature</Source><SourceDirection>+Z</SourceDirection><FeatureName>segment 159</FeatureName></PrimaryAxis><SecondaryAxis><DefinedDirection>+X</DefinedDirection><Source>ReferenceFrame</Source><SourceDirection>+X</SourceDirection><FeatureName></FeatureName></SecondaryAxis></Value></Frame><Frame><Id>Frame2</Id><Value><Name>D22</Name><Origin><Source>GeometricFeature</Source><FeatureName>planar surface 154</FeatureName></Origin><PrimaryAxis><DefinedDirection>+Z</DefinedDirection><Source>ReferenceFrame</Source><SourceDirection>+Z</SourceDirection><FeatureName></FeatureName></PrimaryAxis><SecondaryAxis><DefinedDirection>+X</DefinedDirection><Source>ReferenceFrame</Source><SourceDirection>+X</SourceDirection><FeatureName></FeatureName></SecondaryAxis></Value></Frame></Frames>  GraphicType=FromGeometry  MarkerShape=Sphere  MarkerSize=10  GraphicVisPropType=SimpleVisualProperties  GraphicDiffuseColor=[255 9 134]/255  GraphicSpecularColor=[0.5 0.5 0.5 1.0]  GraphicAmbientColor=[0.15 0.15 0.15 1.0]  GraphicEmissiveColor=[0.0 0.0 0.0 1.0]  GraphicShininess=75  GraphicOpacity=1.0
  P32p_to_P32 : sm_lib/Frames and Transforms/Rigid Transform  TranslationMethod=StandardAxis  TranslationStandardOffset=17  TranslationLengthUnit=mm  TranslationStandardAxis=+Z  TranslationCartesianOffset=[0 0 0]  TranslationROffset=0  TranslationROffsetUnits=m  TranslationZOffset=0  TranslationZOffsetUnits=m  TranslationThetaOffset=0  TranslationThetaOffsetUnits=deg  RotationMethod=None  RotationAngleUnits=deg  RotationStandardAxis=+Y  RotationAngle=-90  RotationArbitraryAxis=[0 0 1]  FollAlignAxisA=+X  BaseAlignAxisA=+Y  FollAlignAxisB=+Y  BaseAlignAxisB=+Z  RotationSequenceAxes=FollowerAxes  RotationSequence=XYX  RotationSequenceAngles=[0 0 0]  RotationSequenceAnglesUnits=deg  RotationMatrix=[1 0 0; 0 1 0; 0 0 1]
  P32 : PMIOPort  Side=Left
  D22 : PMIOPort  Port=2  Side=Left
  connections:
  EndObjectMass/LConn1 -- P32p_to_P32/LConn1
  P32p_to_P32/RConn1 -- P32/RConn1
  D22/RConn1 -- EndObjectMass/RConn1

== system SimForces2022a/sbHydraulicManipulatorSimscape/sbLiftCylinderAndLiftPiston ==
  B31p_to_B31pAux : sm_lib/Frames and Transforms/Rigid Transform  TranslationMethod=None  TranslationStandardOffset=0  TranslationLengthUnit=m  TranslationStandardAxis=+Z  TranslationCartesianOffset=[0 0 0]  TranslationROffset=0  TranslationROffsetUnits=m  TranslationZOffset=0  TranslationZOffsetUnits=m  TranslationThetaOffset=0  TranslationThetaOffsetUnits=deg  RotationMethod=StandardAxis  RotationAngleUnits=deg  RotationStandardAxis=+Y  RotationAngle=90  RotationArbitraryAxis=[0 0 1]  FollAlignAxisA=+X  BaseAlignAxisA=+Y  FollAlignAxisB=+Y  BaseAlignAxisB=+Z  RotationSequenceAxes=FollowerAxes  RotationSequence=XYX  RotationSequenceAngles=[0 0 0]  RotationSequenceAnglesUnits=deg  RotationMatrix=[1 0 0; 0 1 0; 0 0 1]
  B41Aux_to_B41 : sm_lib/Frames and Transforms/Rigid Transform  TranslationMethod=None  TranslationStandardOffset=0  TranslationLengthUnit=m  TranslationStandardAxis=+Z  TranslationCartesianOffset=[0 0 0]  TranslationROffset=0  TranslationROffsetUnits=m  TranslationZOffset=0  TranslationZOffsetUnits=m  TranslationThetaOffset=0  TranslationThetaOffsetUnits=deg  RotationMethod=StandardAxis  RotationAngleUnits=deg  RotationStandardAxis=+Y  RotationAngle=-90  RotationArbitraryAxis=[0 0 1]  FollAlignAxisA=+X  BaseAlignAxisA=+Y  FollAlignAxisB=+Y  BaseAlignAxisB=+Z  RotationSequenceAxes=FollowerAxes  RotationSequence=XYX  RotationSequenceAngles=[0 0 0]  RotationSequenceAnglesUnits=deg  RotationMatrix=[1 0 0; 0 1 0; 0 0 1]
  LiftCylinderSolid : sm_lib/Body Elements/File Solid  ExtGeomFileName=03_LiftCylGP.STEP  UnitType=FromFile  ExtGeomFileUnits=m  StepReaderType=OCC  ExportConvexHullGeometry=off  InertiaType=Custom  Mass=17.36281648  MassUnits=kg  CenterOfMass=[0 0.31781210 0]  CenterOfMassUnits=m  MomentsOfInertia=[0.90735702 0.03150902 0.90763033]  MomentsOfInertiaUnits=kg*m^2  ProductsOfInertia=[0 0 0]  ProductsOfInertiaUnits=kg*m^2  BasedOnType=Density  Density=7300  DensityUnits=kg/m^3  DoExposeReferenceFrame=off  SerializedFrames=<Frames><Frame><Id>Frame1</Id><Value><Name>B31</Name><Origin><Source>GeometricFeature</Source><FeatureName>cylindrical surface 11</FeatureName></Origin><PrimaryAxis><DefinedDirection>+X</DefinedDirection><Source>ReferenceFrame</Source><SourceDirection>+Y</SourceDirection><FeatureName></FeatureName></PrimaryAxis><SecondaryAxis><DefinedDirection>+Y</DefinedDirection><Source>ReferenceFrame</Source><SourceDirection>-X</SourceDirection><FeatureName></FeatureName></SecondaryAxis></Value></Frame><Frame><Id>Frame2</Id><Value><Name>B31p</Name><Origin><Source>GeometricFeature</Source><FeatureName>planar surface 4</FeatureName></Origin><PrimaryAxis><DefinedDirection>+X</DefinedDirection><Source>ReferenceFrame</Source><SourceDirection>+Y</SourceDirection><FeatureName></FeatureName></PrimaryAxis><SecondaryAxis><DefinedDirection>+Y</DefinedDirection><Source>ReferenceFrame</Source><SourceDirection>-X</SourceDirection><FeatureName></FeatureName></SecondaryAxis></Value></Frame></Frames>  GraphicType=FromGeometry  MarkerShape=Sphere  MarkerSize=10  GraphicVisPropType=SimpleVisualProperties  GraphicDiffuseColor=[1 1 119]/255  GraphicSpecularColor=[0.5 0.5 0.5 1.0]  GraphicAmbientColor=[0.15 0.15 0.15 1.0]  GraphicEmissiveColor=[0.0 0.0 0.0 1.0]  GraphicShininess=75  GraphicOpacity=1.0
  LiftPistonSolid : sm_lib/Body Elements/File Solid  ExtGeomFileName=04_LiftPistGP.STEP  UnitType=FromFile  ExtGeomFileUnits=m  StepReaderType=OCC  ExportConvexHullGeometry=off  InertiaType=Custom  Mass=10.34519231  MassUnits=kg  CenterOfMass=[0 0.32981882 0]  CenterOfMassUnits=m  MomentsOfInertia=[0.55759812 0.00370720 0.55785997]  MomentsOfInertiaUnits=kg*m^2  ProductsOfInertia=[0 0 0]  ProductsOfInertiaUnits=kg*m^2  BasedOnType=Density  Density=7800  DensityUnits=kg/m^3  DoExposeReferenceFrame=off  SerializedFrames=<Frames><Frame><Id>Frame2</Id><Value><Name>B41</Name><Origin><Source>GeometricFeature</Source><FeatureName>planar surface 2</FeatureName></Origin><PrimaryAxis><DefinedDirection>+X</DefinedDirection><Source>ReferenceFrame</Source><SourceDirection>+Y</SourceDirection><FeatureName></FeatureName></PrimaryAxis><SecondaryAxis><DefinedDirection>+Y</DefinedDirection><Source>ReferenceFrame</Source><SourceDirection>-X</SourceDirection><FeatureName></FeatureName></SecondaryAxis></Value></Frame><Frame><Id>Frame3</Id><Value><Name>P11</Name><Origin><Source>GeometricFeature</Source><FeatureName>cylindrical surface 8</FeatureName></Origin><PrimaryAxis><DefinedDirection>+X</DefinedDirection><Source>ReferenceFrame</Source><SourceDirection>+Y</SourceDirection><FeatureName></FeatureName></PrimaryAxis><SecondaryAxis><DefinedDirection>+Y</DefinedDirection><Source>ReferenceFrame</Source><SourceDirection>-X</SourceDirection><FeatureName></FeatureName></SecondaryAxis></Value></Frame></Frames>  GraphicType=FromGeometry  MarkerShape=Sphere  MarkerSize=10  GraphicVisPropType=SimpleVisualProperties  GraphicDiffuseColor=[9 232 232]/255  GraphicSpecularColor=[0.5 0.5 0.5 1.0]  GraphicAmbientColor=[0.15 0.15 0.15 1.0]  GraphicEmissiveColor=[0.0 0.0 0.0 1.0]  GraphicShininess=75  GraphicOpacity=1.0
  PS-Sim1 : nesl_utility/PS-Simulink Converter  PhysicalDomain=network_engine_domain  SubClassName=ps_output  LeftPortType=input  RightPortType=output  PseudoPeriodic=off  Frequencies=[]  VectorFormat=1-D array  Unit=inherit  AffineConversion=off
      settings: SourceProductBaseCode=SS,PW,VE
  q11Rotation : sm_lib/Joints/Revolute Joint  JointMode=Normal  SenseConstraintForce=off  SenseConstraintForceX=off  SenseConstraintForceY=off  SenseConstraintForceZ=off  SenseConstraintTorque=off  SenseConstraintTorqueX=off  SenseConstraintTorqueY=off  SenseConstraintTorqueZ=off  SenseTotalForce=off  SenseTotalForceX=off  SenseTotalForceY=off  SenseTotalForceZ=off  SenseTotalTorque=off  SenseTotalTorqueX=off  SenseTotalTorqueY=off  SenseTotalTorqueZ=off  CompositeWrenchDir=FollowerOnBase  CompositeWrenchFrame=BaseFrame  EquilibriumPosition=0  EquilibriumPositionUnits=rad  SpringStiffness=0  SpringStiffnessUnits=N*m/rad  DampingCoefficient=0  DampingCoefficientUnits=N*m/(rad/s)  TorqueActuationMode=NoTorque  MotionActuationMode=ComputedMotion  SensePosition=off  SenseVelocity=off  SenseAcceleration=off  SenseTorqueForce=off  SenseLowerLimitTorqueForce=off  SenseUpperLimitTorqueForce=off  LowerLimitSpecify=off  LowerLimitBound=-90  LowerLimitBoundUnits=deg  LowerLimitStiffness=1e4  LowerLimitStiffnessUnits=N*m/deg  LowerLimitDamping=10  LowerLimitDampingUnits=N*m/(deg/s)  LowerLimitTransitionRegionWidth=0.1  LowerLimitTransitionRegionWidthUnits=deg  UpperLimitSpecify=off  UpperLimitBound=90  UpperLimitBoundUnits=deg  UpperLimitStiffness=1e4  UpperLimitStiffnessUnits=N*m/deg  UpperLimitDamping=10  UpperLimitDampingUnits=N*m/(deg/s)  UpperLimitTransitionRegionWidth=0.1  UpperLimitTransitionRegionWidthUnits=deg  PositionTargetSpecify=off  PositionTargetPriority=High  PositionTargetValue=0  PositionTargetValueUnits=deg  VelocityTargetSpecify=off  VelocityTargetPriority=High  VelocityTargetValue=0  VelocityTargetValueUnits=deg/s
  q12Rotation : sm_lib/Joints/Revolute Joint  JointMode=Normal  SenseConstraintForce=off  SenseConstraintForceX=off  SenseConstraintForceY=off  SenseConstraintForceZ=off  SenseConstraintTorque=off  SenseConstraintTorqueX=off  SenseConstraintTorqueY=off  SenseConstraintTorqueZ=off  SenseTotalForce=off  SenseTotalForceX=off  SenseTotalForceY=off  SenseTotalForceZ=off  SenseTotalTorque=off  SenseTotalTorqueX=off  SenseTotalTorqueY=off  SenseTotalTorqueZ=off  CompositeWrenchDir=FollowerOnBase  CompositeWrenchFrame=BaseFrame  EquilibriumPosition=0  EquilibriumPositionUnits=rad  SpringStiffness=0  SpringStiffnessUnits=N*m/rad  DampingCoefficient=0  DampingCoefficientUnits=N*m/(rad/s)  TorqueActuationMode=NoTorque  MotionActuationMode=ComputedMotion  SensePosition=off  SenseVelocity=off  SenseAcceleration=off  SenseTorqueForce=off  SenseLowerLimitTorqueForce=off  SenseUpperLimitTorqueForce=off  LowerLimitSpecify=off  LowerLimitBound=-90  LowerLimitBoundUnits=deg  LowerLimitStiffness=1e4  LowerLimitStiffnessUnits=N*m/deg  LowerLimitDamping=10  LowerLimitDampingUnits=N*m/(deg/s)  LowerLimitTransitionRegionWidth=0.1  LowerLimitTransitionRegionWidthUnits=deg  UpperLimitSpecify=off  UpperLimitBound=90  UpperLimitBoundUnits=deg  UpperLimitStiffness=1e4  UpperLimitStiffnessUnits=N*m/deg  UpperLimitDamping=10  UpperLimitDampingUnits=N*m/(deg/s)  UpperLimitTransitionRegionWidth=0.1  UpperLimitTransitionRegionWidthUnits=deg  PositionTargetSpecify=off  PositionTargetPriority=High  PositionTargetValue=0  PositionTargetValueUnits=deg  VelocityTargetSpecify=off  VelocityTargetPriority=High  VelocityTargetValue=0  VelocityTargetValueUnits=deg/s
  x1-translation : sm_lib/Joints/Prismatic Joint  JointMode=Normal  SenseConstraintForce=off  SenseConstraintForceX=off  SenseConstraintForceY=off  SenseConstraintForceZ=off  SenseConstraintTorque=off  SenseConstraintTorqueX=off  SenseConstraintTorqueY=off  SenseConstraintTorqueZ=off  SenseTotalForce=off  SenseTotalForceX=off  SenseTotalForceY=off  SenseTotalForceZ=off  SenseTotalTorque=off  SenseTotalTorqueX=off  SenseTotalTorqueY=off  SenseTotalTorqueZ=off  CompositeWrenchDir=FollowerOnBase  CompositeWrenchFrame=FollowerFrame  EquilibriumPosition=0  EquilibriumPositionUnits=m  SpringStiffness=0  SpringStiffnessUnits=N/m  DampingCoefficient=0  DampingCoefficientUnits=N/(m/s)  TorqueActuationMode=ComputedTorque  MotionActuationMode=ComputedMotion  SensePosition=off  SenseVelocity=off  SenseAcceleration=off  SenseTorqueForce=on  SenseLowerLimitTorqueForce=off  SenseUpperLimitTorqueForce=off  LowerLimitSpecify=on  LowerLimitBound=0  LowerLimitBoundUnits=m  LowerLimitStiffness=1e6  LowerLimitStiffnessUnits=N/m  LowerLimitDamping=1e3  LowerLimitDampingUnits=N/(m/s)  LowerLimitTransitionRegionWidth=1e-4  LowerLimitTransitionRegionWidthUnits=m  UpperLimitSpecify=on  UpperLimitBound=cyl1.sp  UpperLimitBoundUnits=m  UpperLimitStiffness=1e6  UpperLimitStiffnessUnits=N/m  UpperLimitDamping=1e3  UpperLimitDampingUnits=N/(m/s)  UpperLimitTransitionRegionWidth=1e-4  UpperLimitTransitionRegionWidthUnits=m  PositionTargetSpecify=on  PositionTargetPriority=Low  PositionTargetValue=0.4  PositionTargetValueUnits=m  VelocityTargetSpecify=on  VelocityTargetPriority=High  VelocityTargetValue=0  VelocityTargetValueUnits=m/s
  B31 : PMIOPort  Side=Left
  B41 : PMIOPort  Port=2  Side=Left
  F1 : PMIOPort  Port=3  Side=Right
  F3 : PMIOPort  Port=4  Side=Right
  fc1 : Outport
  wires:
  PS-Sim1/1 -> fc1/1
  connections:
  B31p_to_B31pAux/LConn1 -- LiftCylinderSolid/RConn1
  x1-translation/RConn1 -- B41Aux_to_B41/LConn1
  q11Rotation/RConn1 -- B31/RConn1 -- LiftCylinderSolid/LConn1
  LiftPistonSolid/LConn1 -- B41/RConn1 -- B41Aux_to_B41/RConn1
  B31p_to_B31pAux/RConn1 -- x1-translation/LConn1
  q11Rotation/LConn1 -- F1/RConn1
  q12Rotation/LConn1 -- LiftPistonSolid/RConn1
  q12Rotation/RConn1 -- F3/RConn1
  PS-Sim1/LConn1 -- x1-translation/RConn2
